simulink model "ejercicio_2_05_10_jevg"  (R2021a)
settings: Solver=VariableStepAuto  StartTime=0.0  StopTime=10.0  RelTol=1e-3
libraries: fl_lib x10, nesl_utility x7
settings Model: Creator=luiss  LastModifiedBy=user
settings DebuggingCC: UnconnectedInputMsg=none  UnconnectedOutputMsg=none  UnconnectedLineMsg=none
settings ModelReferenceCC: EnableRefExpFcnMdlSchedulingChecks=off
settings RTWCC: Description=Generic Real-Time Target  DLArmComputeVersion=20.02.1

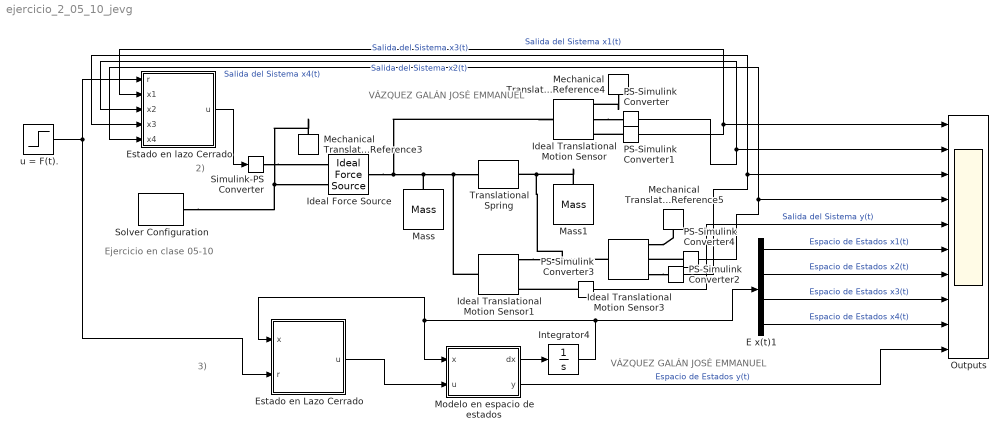
== system ejercicio_2_05_10_jevg ==
  note: Ejercicio en clase
      | 05-10
  note: 3)
  note: 2)
  note: VÁZQUEZ GALÁN JOSÉ EMMANUEL
  note: VÁZQUEZ GALÁN JOSÉ EMMANUEL
  E x(t)1 : Demux
  Estado en Lazo Cerrado : MATLAB Function  TreatAsAtomicUnit=on
  Estado en lazo Cerrado : MATLAB Function  TreatAsAtomicUnit=on
  Ideal Force Source : fl_lib/Mechanical/Mechanical Sources/Ideal Force Source
  Ideal Translational Motion Sensor : fl_lib/Mechanical/Mechanical Sensors/Ideal Translational Motion Sensor  offset=0 m
  Ideal Translational Motion Sensor1 : fl_lib/Mechanical/Mechanical Sensors/Ideal Translational Motion Sensor  offset=0 m
  Ideal Translational Motion Sensor3 : fl_lib/Mechanical/Mechanical Sensors/Ideal Translational Motion Sensor  offset=0 m
  Integrator4 : Integrator  InitialCondition=[0;0;0;0]
  Mass : fl_lib/Mechanical/Translational Elements/Mass  mass=1 kg  num_ports=foundation.enum.numPorts2.one  v_specify=off  v_priority=High  v=0 m/s  v_nominal_specify=off  v_nominal_unit=m/s  v_nominal_value=1  f_specify=off  f_priority=None  f=0 N  f_nominal_specify=off  f_nominal_unit=N  f_nominal_value=1
  Mass1 : fl_lib/Mechanical/Translational Elements/Mass  mass=1 kg  num_ports=foundation.enum.numPorts2.one  v_specify=off  v_priority=High  v=0 m/s  v_nominal_specify=off  v_nominal_unit=m/s  v_nominal_value=1  f_specify=off  f_priority=None  f=0 N  f_nominal_specify=off  f_nominal_unit=N  f_nominal_value=1
  Mechanical Translational Reference3 : fl_lib/Mechanical/Translational Elements/Mechanical Translational Reference
  Mechanical Translational Reference4 : fl_lib/Mechanical/Translational Elements/Mechanical Translational Reference
  Mechanical Translational Reference5 : fl_lib/Mechanical/Translational Elements/Mechanical Translational Reference
  Modelo en espacio de estados : MATLAB Function  TreatAsAtomicUnit=on
  Outputs : Scope  NumInputPorts=10
  PS-Simulink Converter{,1..4} (5 alike) : nesl_utility/PS-Simulink Converter  PhysicalDomain=network_engine_domain  SubClassName=ps_output  LeftPortType=input  RightPortType=output  PseudoPeriodic=off  Frequencies=[]  Unit=inherit  AffineConversion=off
      settings: SourceProductBaseCode=PW,SS
  Simulink-PS Converter : nesl_utility/Simulink-PS Converter  PhysicalDomain=network_engine_domain  SubClassName=ps_input  LeftPortType=input  RightPortType=output  PseudoPeriodic=off  Frequencies=[]  NoiseDistribution=none  NoiseParameters=[]  Unit=1  AffineConversion=off  FilteringAndDerivatives=provide  SimscapeFilterOrder=1  InputFilterTimeConstant=0.001  UdotUserProvided=0
      settings: SourceProductBaseCode=PW,SS
  Solver Configuration : nesl_utility/Solver Configuration  PhysicalDomain=network_engine_domain  SubClassName=solver  LeftPortType=input  RightPortType=generic  Tones=[]  Harmonics=[]  SimulateNoise=off  Profile=off  UseLocalSampling=off  EnableSwitchedLinearOptims=on  FrequencyDomain=off  UseCCode=off  RelTol=0.001  AbsTol=0.001  MinStep=1e-09  ToWorkspace=off  RevertToSquareIcSolve=off  NumHomotopyIterations=100  PhasorMode=off  PhasorModeNumHarmonics=1  DoDC=off  ResidualTolerance=1e-09  UseLocalSolver=off  LocalSolverChoice=NE_BACKWARD_EULER_ADVANCER  LocalSolverSampleTime=0.001  DoFixedCost=off  MaxNonlinIter=3  MaxModeIter=2  ComputeImpulses=off  ImpulseIterations=2  LinearAlgebra=auto  EquationFormulation=NE_TIME_EF  DelaysMemoryBudget=1024  AutomaticFiltering=on  FilteringTimeConstant=0.001  PartitionStorageMethod=AS_NEEDED  PartitionMemoryBudget=1024  PartitionMethod=ROBUST
      settings: SourceProductBaseCode=PW,SS
  Translational Spring : fl_lib/Mechanical/Translational Elements/Translational Spring  spr_rate=1 N/m  v_specify=off  v_priority=None  v=0 m/s  v_nominal_specify=off  v_nominal_unit=m/s  v_nominal_value=1  f_specify=off  f_priority=None  f=0 N  f_nominal_specify=off  f_nominal_unit=N  f_nominal_value=1  x_specify=off  x_priority=High  x=0 m  x_nominal_specify=off  x_nominal_unit=m  x_nominal_value=1
  "u = F(t). " : Step  SampleTime=0
  wires:
  Integrator4/1 -> Estado en Lazo Cerrado/1(x), Modelo en espacio de estados/1(x), E x(t)1/1
  Modelo en espacio de estados/1(dx) -> Integrator4/1
  Modelo en espacio de estados/2(y) -> Outputs/10  "Espacio de Estados y(t)"
  PS-Simulink Converter3/1 -> Outputs/5  "Salida del Sistema y(t)"
  PS-Simulink Converter2/1 -> Estado en lazo Cerrado/4(x3), Outputs/3  "Salida del Sistema x3(t)"
  PS-Simulink Converter/1 -> Estado en lazo Cerrado/3(x2), Outputs/2  "Salida del Sistema x2(t)"
  PS-Simulink Converter1/1 -> Estado en lazo Cerrado/2(x1), Outputs/1  "Salida del Sistema x1(t)"
  E x(t)1/3 -> Outputs/8  "Espacio de Estados x3(t)"
  E x(t)1/1 -> Outputs/6  "Espacio de Estados x1(t)"
  E x(t)1/2 -> Outputs/7  "Espacio de Estados x2(t)"
  "u = F(t). "/1 -> Estado en lazo Cerrado/1(r), Estado en Lazo Cerrado/2(r)
  PS-Simulink Converter4/1 -> Estado en lazo Cerrado/5(x4), Outputs/4  "Salida del Sistema x4(t)"
  Estado en lazo Cerrado/1(u) -> Simulink-PS Converter/1
  Estado en Lazo Cerrado/1(u) -> Modelo en espacio de estados/2(u)
  E x(t)1/4 -> Outputs/9  "Espacio de Estados x4(t)"
  connections:
  Ideal Translational Motion Sensor/LConn1 -- Ideal Force Source/LConn1 -- Ideal Translational Motion Sensor1/LConn1 -- Translational Spring/LConn1 -- Mass/LConn1
  Simulink-PS Converter/RConn1 -- Ideal Force Source/RConn1
  Mechanical Translational Reference3/LConn1 -- Solver Configuration/RConn1 -- Ideal Force Source/RConn2
  Ideal Translational Motion Sensor3/LConn1 -- Ideal Translational Motion Sensor1/RConn1 -- Mass1/LConn1 -- Translational Spring/RConn1
  Mechanical Translational Reference4/LConn1 -- Ideal Translational Motion Sensor/RConn1
  Ideal Translational Motion Sensor3/RConn1 -- Mechanical Translational Reference5/LConn1
  PS-Simulink Converter1/LConn1 -- Ideal Translational Motion Sensor/RConn3
  Ideal Translational Motion Sensor/RConn2 -- PS-Simulink Converter/LConn1
  Ideal Translational Motion Sensor3/RConn3 -- PS-Simulink Converter2/LConn1
  PS-Simulink Converter3/LConn1 -- Ideal Translational Motion Sensor1/RConn3
  PS-Simulink Converter4/LConn1 -- Ideal Translational Motion Sensor3/RConn2

== matlab function ejercicio_2_05_10_jevg/Estado en lazo Cerrado ==
  data: r input; u output; x1 input; x2 input; x3 input; x4 input
function u = fcn(r,x1,x2,x3,x4)
% Esta función calcula el control u basado en la entrada r y el estado actual del sistema x.

% Definiendo la matriz de ganancias K
K = [60 12 65 128];

% Organizando las variables de estado en un vector columna
x = [x1,x2,x3,x4]';

% Calculando la señal de control u usando la retroalimentación de estado
u = r - K*x;

== matlab function ejercicio_2_05_10_jevg/Estado en Lazo Cerrado ==
  data: x input; r input; u output
function u = fcn(x,r)
% Esta función calcula el control u basado en la entrada r y el estado actual del sistema x (como vector).

% Definiendo la matriz de ganancias K
K = [60 12 65 128];

% Calculando la señal de control u usando la retroalimentación de estado
u = r - K*x;

== matlab function ejercicio_2_05_10_jevg/Modelo en espacio de estados ==
  data: x input; dx output; u input; y output
function [dx,y] = fcn(x,u)
% Esta función calcula la derivada del estado dx y la salida y basado en el estado actual x y la señal de control u.

% Definiendo constantes y parámetros del sistema
m1 = 1;
m2 = 1;
k = 1;


% Definiendo la matriz A del sistema en el espacio de estados
A = [0  1  0  0; 
    (-k/m1)  0  (k/m1)  0;
     0  0  0  1;
     (k/m2)  0  (-k/m2)  0];
% Definiendo la matriz B del sistema en el espacio de estados
B = [0; 
    1/m1; 
    0;
    0];

% Definiendo la matriz C para la salida
C = [1 0 -1 0];

% Calculando la derivada del estado
dx = A*x + B*u;

% Calculando la salida
y = C*x;
